simulink model "vjezbe_7_5"  (R2017b)
settings: Solver=VariableStepAuto  StartTime=0.0  StopTime=800  RelTol=1e-3
undefined symbols (not defined in the file): ln
libraries: simulink x14
settings Model: Creator=Sead  LastModifiedBy=Sead

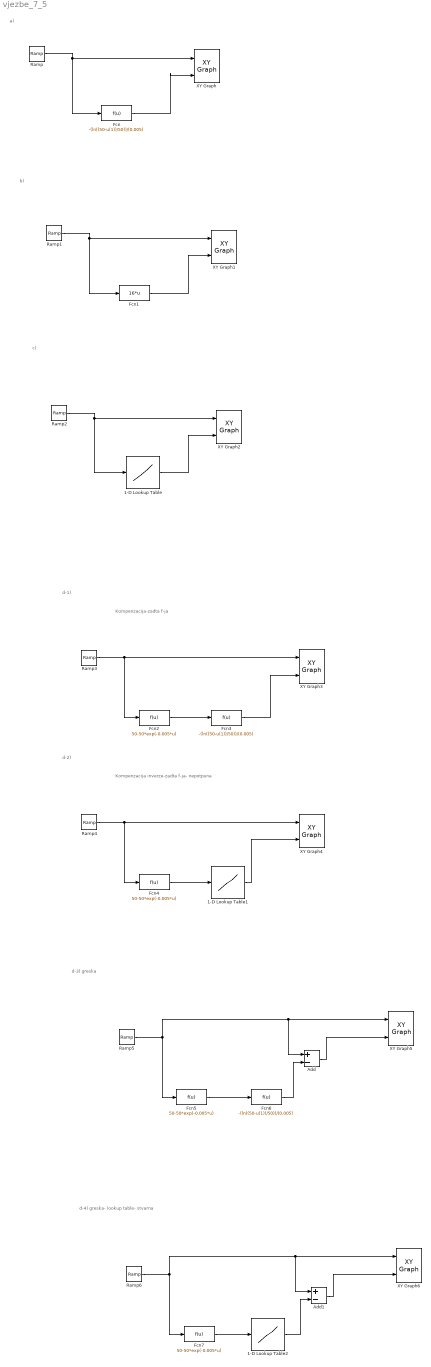
== system vjezbe_7_5 ==
  note: d-3) greska
  note: Kompenzacija-zadta f-ja
  note: a)
  note: b)
  note: c)
  note: d-1)
  note: Kompenzacija inverze-zadta f-ja- nepotpuna
  note: d-2)
  note: d-4) greska- lookup table- stvarna
  1-D Lookup Table : Lookup_n-D  NumberOfTableDimensions=1  BreakpointsForDimension1=50-50*exp(-0.005*[0:100:800])  Table=[0:100:800]  InternalRulePriority=Speed  RndMeth=Simplest  InputSameDT=on
  1-D Lookup Table1 : Lookup_n-D  NumberOfTableDimensions=1  BreakpointsForDimension1=50-50*exp(-0.005*[0:100:800])  Table=[0:100:800]  InternalRulePriority=Speed  RndMeth=Simplest  InputSameDT=on
  1-D Lookup Table2 : Lookup_n-D  NumberOfTableDimensions=1  BreakpointsForDimension1=50-50*exp(-0.005*[0:100:800])  Table=[0:100:800]  InternalRulePriority=Speed  RndMeth=Simplest  InputSameDT=on
  Add : Sum  Inputs=+-
  Add1 : Sum  Inputs=+-
  Fcn : Fcn  Expr=-(ln((50-u(1))/50))/(0.005)
  Fcn1 : Fcn  Expr=16*u
  Fcn{2,4..5,7} (4 alike) : Fcn  Expr=50-50*exp(-0.005*u)
  Fcn3 : Fcn  Expr=-(ln((50-u(1))/50))/(0.005)
  Fcn6 : Fcn  Expr=-(ln((50-u(1))/50))/(0.005)
  Ramp{,1..6} (7 alike) : simulink/Sources/Ramp  slope=1  start=0  X0=0
  XY Graph : simulink/Sinks/XY Graph  xmin=0  xmax=50  ymin=0  ymax=800  st=1
  XY Graph1 : simulink/Sinks/XY Graph  xmin=0  xmax=50  ymin=0  ymax=800  st=1
  XY Graph2 : simulink/Sinks/XY Graph  xmin=0  xmax=50  ymin=0  ymax=800  st=1
  XY Graph3 : simulink/Sinks/XY Graph  xmin=0  xmax=800  ymin=0  ymax=800  st=1
  XY Graph4 : simulink/Sinks/XY Graph  xmin=0  xmax=800  ymin=0  ymax=800  st=1
  XY Graph5 : simulink/Sinks/XY Graph  xmin=0  xmax=800  ymin=-0.01  ymax=0.01  st=1
  XY Graph6 : simulink/Sinks/XY Graph  xmin=0  xmax=800  ymin=-10  ymax=10  st=1
  wires:
  Fcn/1 -> XY Graph/2
  Ramp/1 -> Fcn/1, XY Graph/1
  Ramp1/1 -> XY Graph1/1, Fcn1/1
  Fcn1/1 -> XY Graph1/2
  1-D Lookup Table/1 -> XY Graph2/2
  Ramp2/1 -> 1-D Lookup Table/1, XY Graph2/1
  Ramp3/1 -> Fcn2/1, XY Graph3/1
  Fcn3/1 -> XY Graph3/2
  Fcn2/1 -> Fcn3/1
  Fcn4/1 -> 1-D Lookup Table1/1
  1-D Lookup Table1/1 -> XY Graph4/2
  Ramp4/1 -> XY Graph4/1, Fcn4/1
  Ramp5/1 -> Fcn5/1, Add/1, XY Graph5/1
  Add/1 -> XY Graph5/2
  Fcn5/1 -> Fcn6/1
  Fcn6/1 -> Add/2
  1-D Lookup Table2/1 -> Add1/2
  Fcn7/1 -> 1-D Lookup Table2/1
  Add1/1 -> XY Graph6/2
  Ramp6/1 -> XY Graph6/1, Add1/1, Fcn7/1
